simulink model "RigidJoint_Adaptive_PD"  (R2019b)
settings: Solver=VariableStepAuto  StartTime=0.0  StopTime=10  RelTol=1e-3
libraries: simulink x6
settings Model: Creator=USER  LastModifiedBy=USER

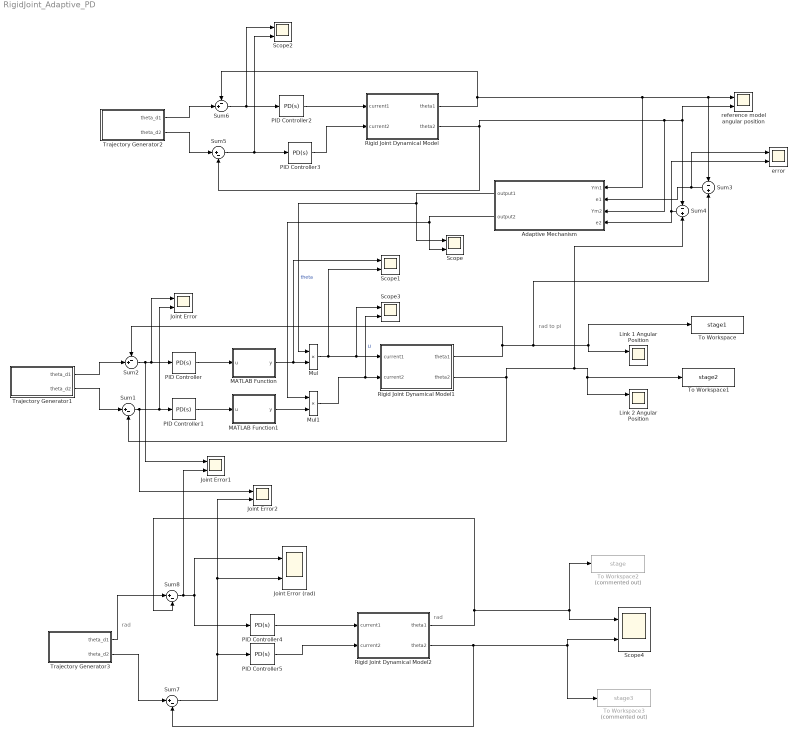
== system RigidJoint_Adaptive_PD ==
  note: rad to pi
  note: rad
  note: rad
  Adaptive Mechanism : Subsystem
  Joint Error : Scope  NumInputPorts=2
  Joint Error (rad) : Scope  NumInputPorts=2
  Joint Error1 : Scope  NumInputPorts=2
  Joint Error2 : Scope  NumInputPorts=2
  Link 1 Angular Position : Scope  NumInputPorts=2
  Link 2 Angular Position : Scope  NumInputPorts=2
  MATLAB Function : MATLAB Function  TreatAsAtomicUnit=on
  MATLAB Function1 : MATLAB Function  TreatAsAtomicUnit=on
  Mul : Product
  Mul1 : Product
  PID Controller : simulink/Continuous/PID Controller  Controller=PD  Form=Parallel  TimeDomain=Continuous-time  SampleTime=-1  IntegratorMethod=Forward Euler  FilterMethod=Forward Euler  ControllerParametersSource=internal  P=3  I=0.00248207984793386  D=0.6  UseFilter=on  N=100  TunerSelectOption=Transfer Function Based (PID Tuner App)  InitialConditionSource=internal  InitialConditionForIntegrator=0  InitialConditionForFilter=0  DifferentiatorICPrevScaledInput=0  ExternalReset=none  TrackingMode=off  Kt=1  LimitOutput=off  UpperSaturationLimit=inf  LowerSaturationLimit=-inf  LinearizeAsGain=on  AntiWindupMode=none  Kb=1  POutMin=[]  POutMax=[]  IOutMin=[]  IOutMax=[]  DOutMin=[]  DOutMax=[]  NOutMin=[]  NOutMax=[]  SumOutMin=[]  SumOutMax=[]  SaturationOutMin=[]  SaturationOutMax=[]  PParamMin=[]  PParamMax=[]  IParamMin=[]  IParamMax=[]  DParamMin=[]  DParamMax=[]  NParamMin=[]  NParamMax=[]  KbParamMin=[]  KbParamMax=[]  KtParamMin=[]  KtParamMax=[]  KbOutMin=[]  KbOutMax=[]  KtOutMin=[]  KtOutMax=[]  IntegratorOutMin=[]  IntegratorOutMax=[]  FilterOutMin=[]  FilterOutMax=[]  SumI1OutMin=[]  SumI1OutMax=[]  SumI2OutMin=[]  SumI2OutMax=[]  SumI3OutMin=[]  SumI3OutMax=[]  SumI4OutMin=[]  SumI4OutMax=[]  SumDOutMin=[]  SumDOutMax=[]  DifferentiatorOutMin=[]  DifferentiatorOutMax=[]  FilterDiffOutCoefMin=[]  FilterDiffOutCoefMax=[]  ReciprocalOutMin=[]  ReciprocalOutMax=[]  SumDenOutMin=[]  SumDenOutMax=[]  SumNumOutMin=[]  SumNumOutMax=[]  DivideOutMin=[]  DivideOutMax=[]  IntegratorContinuousStateAttributes=''  IntegratorStateMustResolveToSignalObject=off  IntegratorRTWStateStorageClass=Auto  FilterContinuousStateAttributes=''  FilterStateMustResolveToSignalObject=off  FilterRTWStateStorageClass=Auto  ParallelPVariant=InternalParameters  IdealPVariant=Disabled  IVariant=Disabled  DVariant=InternalParameters  IntegratorVariant=Disabled  SatVariant=Disabled  AWVariant=Disabled  PCopyVariant=Disabled  TRVariant=Disabled  FdbkBlocksVariant=Forward  IdealPFdbkVariant=Disabled  SatFdbkVariant=Disabled  DerivativeFilterVariant=ContFilter  NVariant=InternalParameters  NCopyVariant=Disabled  FilterICVariant=InternalICsFilter  IntegratorICVariant=Disabled  ExternalResetVariant=Disabled  TRSumVariant=Passthrough  SumFdbkVariant=Disabled  SumVariant=Sum_PD
  PID Controller1 : simulink/Continuous/PID Controller  Controller=PD  Form=Parallel  TimeDomain=Continuous-time  SampleTime=-1  IntegratorMethod=Forward Euler  FilterMethod=Forward Euler  ControllerParametersSource=internal  P=8  I=0.00248207984793386  D=0.8  UseFilter=on  N=100  TunerSelectOption=Transfer Function Based (PID Tuner App)  InitialConditionSource=internal  InitialConditionForIntegrator=0  InitialConditionForFilter=0  DifferentiatorICPrevScaledInput=0  ExternalReset=none  TrackingMode=off  Kt=1  LimitOutput=off  UpperSaturationLimit=inf  LowerSaturationLimit=-inf  LinearizeAsGain=on  AntiWindupMode=none  Kb=1  POutMin=[]  POutMax=[]  IOutMin=[]  IOutMax=[]  DOutMin=[]  DOutMax=[]  NOutMin=[]  NOutMax=[]  SumOutMin=[]  SumOutMax=[]  SaturationOutMin=[]  SaturationOutMax=[]  PParamMin=[]  PParamMax=[]  IParamMin=[]  IParamMax=[]  DParamMin=[]  DParamMax=[]  NParamMin=[]  NParamMax=[]  KbParamMin=[]  KbParamMax=[]  KtParamMin=[]  KtParamMax=[]  KbOutMin=[]  KbOutMax=[]  KtOutMin=[]  KtOutMax=[]  IntegratorOutMin=[]  IntegratorOutMax=[]  FilterOutMin=[]  FilterOutMax=[]  SumI1OutMin=[]  SumI1OutMax=[]  SumI2OutMin=[]  SumI2OutMax=[]  SumI3OutMin=[]  SumI3OutMax=[]  SumI4OutMin=[]  SumI4OutMax=[]  SumDOutMin=[]  SumDOutMax=[]  DifferentiatorOutMin=[]  DifferentiatorOutMax=[]  FilterDiffOutCoefMin=[]  FilterDiffOutCoefMax=[]  ReciprocalOutMin=[]  ReciprocalOutMax=[]  SumDenOutMin=[]  SumDenOutMax=[]  SumNumOutMin=[]  SumNumOutMax=[]  DivideOutMin=[]  DivideOutMax=[]  IntegratorContinuousStateAttributes=''  IntegratorStateMustResolveToSignalObject=off  IntegratorRTWStateStorageClass=Auto  FilterContinuousStateAttributes=''  FilterStateMustResolveToSignalObject=off  FilterRTWStateStorageClass=Auto  ParallelPVariant=InternalParameters  IdealPVariant=Disabled  IVariant=Disabled  DVariant=InternalParameters  IntegratorVariant=Disabled  SatVariant=Disabled  AWVariant=Disabled  PCopyVariant=Disabled  TRVariant=Disabled  FdbkBlocksVariant=Forward  IdealPFdbkVariant=Disabled  SatFdbkVariant=Disabled  DerivativeFilterVariant=ContFilter  NVariant=InternalParameters  NCopyVariant=Disabled  FilterICVariant=InternalICsFilter  IntegratorICVariant=Disabled  ExternalResetVariant=Disabled  TRSumVariant=Passthrough  SumFdbkVariant=Disabled  SumVariant=Sum_PD
  PID Controller2 : simulink/Continuous/PID Controller  Controller=PD  Form=Parallel  TimeDomain=Continuous-time  SampleTime=-1  IntegratorMethod=Forward Euler  FilterMethod=Forward Euler  ControllerParametersSource=internal  P=3  I=0.00248207984793386  D=0.6  UseFilter=on  N=100  TunerSelectOption=Transfer Function Based (PID Tuner App)  InitialConditionSource=internal  InitialConditionForIntegrator=0  InitialConditionForFilter=0  DifferentiatorICPrevScaledInput=0  ExternalReset=none  TrackingMode=off  Kt=1  LimitOutput=off  UpperSaturationLimit=inf  LowerSaturationLimit=-inf  LinearizeAsGain=on  AntiWindupMode=none  Kb=1  POutMin=[]  POutMax=[]  IOutMin=[]  IOutMax=[]  DOutMin=[]  DOutMax=[]  NOutMin=[]  NOutMax=[]  SumOutMin=[]  SumOutMax=[]  SaturationOutMin=[]  SaturationOutMax=[]  PParamMin=[]  PParamMax=[]  IParamMin=[]  IParamMax=[]  DParamMin=[]  DParamMax=[]  NParamMin=[]  NParamMax=[]  KbParamMin=[]  KbParamMax=[]  KtParamMin=[]  KtParamMax=[]  KbOutMin=[]  KbOutMax=[]  KtOutMin=[]  KtOutMax=[]  IntegratorOutMin=[]  IntegratorOutMax=[]  FilterOutMin=[]  FilterOutMax=[]  SumI1OutMin=[]  SumI1OutMax=[]  SumI2OutMin=[]  SumI2OutMax=[]  SumI3OutMin=[]  SumI3OutMax=[]  SumI4OutMin=[]  SumI4OutMax=[]  SumDOutMin=[]  SumDOutMax=[]  DifferentiatorOutMin=[]  DifferentiatorOutMax=[]  FilterDiffOutCoefMin=[]  FilterDiffOutCoefMax=[]  ReciprocalOutMin=[]  ReciprocalOutMax=[]  SumDenOutMin=[]  SumDenOutMax=[]  SumNumOutMin=[]  SumNumOutMax=[]  DivideOutMin=[]  DivideOutMax=[]  IntegratorContinuousStateAttributes=''  IntegratorStateMustResolveToSignalObject=off  IntegratorRTWStateStorageClass=Auto  FilterContinuousStateAttributes=''  FilterStateMustResolveToSignalObject=off  FilterRTWStateStorageClass=Auto  ParallelPVariant=InternalParameters  IdealPVariant=Disabled  IVariant=Disabled  DVariant=InternalParameters  IntegratorVariant=Disabled  SatVariant=Disabled  AWVariant=Disabled  PCopyVariant=Disabled  TRVariant=Disabled  FdbkBlocksVariant=Forward  IdealPFdbkVariant=Disabled  SatFdbkVariant=Disabled  DerivativeFilterVariant=ContFilter  NVariant=InternalParameters  NCopyVariant=Disabled  FilterICVariant=InternalICsFilter  IntegratorICVariant=Disabled  ExternalResetVariant=Disabled  TRSumVariant=Passthrough  SumFdbkVariant=Disabled  SumVariant=Sum_PD
  PID Controller3 : simulink/Continuous/PID Controller  Controller=PD  Form=Parallel  TimeDomain=Continuous-time  SampleTime=-1  IntegratorMethod=Forward Euler  FilterMethod=Forward Euler  ControllerParametersSource=internal  P=8  I=0.00248207984793386  D=0.8  UseFilter=on  N=100  TunerSelectOption=Transfer Function Based (PID Tuner App)  InitialConditionSource=internal  InitialConditionForIntegrator=0  InitialConditionForFilter=0  DifferentiatorICPrevScaledInput=0  ExternalReset=none  TrackingMode=off  Kt=1  LimitOutput=off  UpperSaturationLimit=inf  LowerSaturationLimit=-inf  LinearizeAsGain=on  AntiWindupMode=none  Kb=1  POutMin=[]  POutMax=[]  IOutMin=[]  IOutMax=[]  DOutMin=[]  DOutMax=[]  NOutMin=[]  NOutMax=[]  SumOutMin=[]  SumOutMax=[]  SaturationOutMin=[]  SaturationOutMax=[]  PParamMin=[]  PParamMax=[]  IParamMin=[]  IParamMax=[]  DParamMin=[]  DParamMax=[]  NParamMin=[]  NParamMax=[]  KbParamMin=[]  KbParamMax=[]  KtParamMin=[]  KtParamMax=[]  KbOutMin=[]  KbOutMax=[]  KtOutMin=[]  KtOutMax=[]  IntegratorOutMin=[]  IntegratorOutMax=[]  FilterOutMin=[]  FilterOutMax=[]  SumI1OutMin=[]  SumI1OutMax=[]  SumI2OutMin=[]  SumI2OutMax=[]  SumI3OutMin=[]  SumI3OutMax=[]  SumI4OutMin=[]  SumI4OutMax=[]  SumDOutMin=[]  SumDOutMax=[]  DifferentiatorOutMin=[]  DifferentiatorOutMax=[]  FilterDiffOutCoefMin=[]  FilterDiffOutCoefMax=[]  ReciprocalOutMin=[]  ReciprocalOutMax=[]  SumDenOutMin=[]  SumDenOutMax=[]  SumNumOutMin=[]  SumNumOutMax=[]  DivideOutMin=[]  DivideOutMax=[]  IntegratorContinuousStateAttributes=''  IntegratorStateMustResolveToSignalObject=off  IntegratorRTWStateStorageClass=Auto  FilterContinuousStateAttributes=''  FilterStateMustResolveToSignalObject=off  FilterRTWStateStorageClass=Auto  ParallelPVariant=InternalParameters  IdealPVariant=Disabled  IVariant=Disabled  DVariant=InternalParameters  IntegratorVariant=Disabled  SatVariant=Disabled  AWVariant=Disabled  PCopyVariant=Disabled  TRVariant=Disabled  FdbkBlocksVariant=Forward  IdealPFdbkVariant=Disabled  SatFdbkVariant=Disabled  DerivativeFilterVariant=ContFilter  NVariant=InternalParameters  NCopyVariant=Disabled  FilterICVariant=InternalICsFilter  IntegratorICVariant=Disabled  ExternalResetVariant=Disabled  TRSumVariant=Passthrough  SumFdbkVariant=Disabled  SumVariant=Sum_PD
  PID Controller4 : simulink/Continuous/PID Controller  Controller=PD  Form=Parallel  TimeDomain=Continuous-time  SampleTime=-1  IntegratorMethod=Forward Euler  FilterMethod=Forward Euler  ControllerParametersSource=internal  P=3  I=0.00248207984793386  D=0.6  UseFilter=on  N=100  TunerSelectOption=Transfer Function Based (PID Tuner App)  InitialConditionSource=internal  InitialConditionForIntegrator=0  InitialConditionForFilter=0  DifferentiatorICPrevScaledInput=0  ExternalReset=none  TrackingMode=off  Kt=1  LimitOutput=off  UpperSaturationLimit=inf  LowerSaturationLimit=-inf  LinearizeAsGain=on  AntiWindupMode=none  Kb=1  POutMin=[]  POutMax=[]  IOutMin=[]  IOutMax=[]  DOutMin=[]  DOutMax=[]  NOutMin=[]  NOutMax=[]  SumOutMin=[]  SumOutMax=[]  SaturationOutMin=[]  SaturationOutMax=[]  PParamMin=[]  PParamMax=[]  IParamMin=[]  IParamMax=[]  DParamMin=[]  DParamMax=[]  NParamMin=[]  NParamMax=[]  KbParamMin=[]  KbParamMax=[]  KtParamMin=[]  KtParamMax=[]  KbOutMin=[]  KbOutMax=[]  KtOutMin=[]  KtOutMax=[]  IntegratorOutMin=[]  IntegratorOutMax=[]  FilterOutMin=[]  FilterOutMax=[]  SumI1OutMin=[]  SumI1OutMax=[]  SumI2OutMin=[]  SumI2OutMax=[]  SumI3OutMin=[]  SumI3OutMax=[]  SumI4OutMin=[]  SumI4OutMax=[]  SumDOutMin=[]  SumDOutMax=[]  DifferentiatorOutMin=[]  DifferentiatorOutMax=[]  FilterDiffOutCoefMin=[]  FilterDiffOutCoefMax=[]  ReciprocalOutMin=[]  ReciprocalOutMax=[]  SumDenOutMin=[]  SumDenOutMax=[]  SumNumOutMin=[]  SumNumOutMax=[]  DivideOutMin=[]  DivideOutMax=[]  IntegratorContinuousStateAttributes=''  IntegratorStateMustResolveToSignalObject=off  IntegratorRTWStateStorageClass=Auto  FilterContinuousStateAttributes=''  FilterStateMustResolveToSignalObject=off  FilterRTWStateStorageClass=Auto  ParallelPVariant=InternalParameters  IdealPVariant=Disabled  IVariant=Disabled  DVariant=InternalParameters  IntegratorVariant=Disabled  SatVariant=Disabled  AWVariant=Disabled  PCopyVariant=Disabled  TRVariant=Disabled  FdbkBlocksVariant=Forward  IdealPFdbkVariant=Disabled  SatFdbkVariant=Disabled  DerivativeFilterVariant=ContFilter  NVariant=InternalParameters  NCopyVariant=Disabled  FilterICVariant=InternalICsFilter  IntegratorICVariant=Disabled  ExternalResetVariant=Disabled  TRSumVariant=Passthrough  SumFdbkVariant=Disabled  SumVariant=Sum_PD
  PID Controller5 : simulink/Continuous/PID Controller  Controller=PD  Form=Parallel  TimeDomain=Continuous-time  SampleTime=-1  IntegratorMethod=Forward Euler  FilterMethod=Forward Euler  ControllerParametersSource=internal  P=8  I=0.00248207984793386  D=0.8  UseFilter=on  N=100  TunerSelectOption=Transfer Function Based (PID Tuner App)  InitialConditionSource=internal  InitialConditionForIntegrator=0  InitialConditionForFilter=0  DifferentiatorICPrevScaledInput=0  ExternalReset=none  TrackingMode=off  Kt=1  LimitOutput=off  UpperSaturationLimit=inf  LowerSaturationLimit=-inf  LinearizeAsGain=on  AntiWindupMode=none  Kb=1  POutMin=[]  POutMax=[]  IOutMin=[]  IOutMax=[]  DOutMin=[]  DOutMax=[]  NOutMin=[]  NOutMax=[]  SumOutMin=[]  SumOutMax=[]  SaturationOutMin=[]  SaturationOutMax=[]  PParamMin=[]  PParamMax=[]  IParamMin=[]  IParamMax=[]  DParamMin=[]  DParamMax=[]  NParamMin=[]  NParamMax=[]  KbParamMin=[]  KbParamMax=[]  KtParamMin=[]  KtParamMax=[]  KbOutMin=[]  KbOutMax=[]  KtOutMin=[]  KtOutMax=[]  IntegratorOutMin=[]  IntegratorOutMax=[]  FilterOutMin=[]  FilterOutMax=[]  SumI1OutMin=[]  SumI1OutMax=[]  SumI2OutMin=[]  SumI2OutMax=[]  SumI3OutMin=[]  SumI3OutMax=[]  SumI4OutMin=[]  SumI4OutMax=[]  SumDOutMin=[]  SumDOutMax=[]  DifferentiatorOutMin=[]  DifferentiatorOutMax=[]  FilterDiffOutCoefMin=[]  FilterDiffOutCoefMax=[]  ReciprocalOutMin=[]  ReciprocalOutMax=[]  SumDenOutMin=[]  SumDenOutMax=[]  SumNumOutMin=[]  SumNumOutMax=[]  DivideOutMin=[]  DivideOutMax=[]  IntegratorContinuousStateAttributes=''  IntegratorStateMustResolveToSignalObject=off  IntegratorRTWStateStorageClass=Auto  FilterContinuousStateAttributes=''  FilterStateMustResolveToSignalObject=off  FilterRTWStateStorageClass=Auto  ParallelPVariant=InternalParameters  IdealPVariant=Disabled  IVariant=Disabled  DVariant=InternalParameters  IntegratorVariant=Disabled  SatVariant=Disabled  AWVariant=Disabled  PCopyVariant=Disabled  TRVariant=Disabled  FdbkBlocksVariant=Forward  IdealPFdbkVariant=Disabled  SatFdbkVariant=Disabled  DerivativeFilterVariant=ContFilter  NVariant=InternalParameters  NCopyVariant=Disabled  FilterICVariant=InternalICsFilter  IntegratorICVariant=Disabled  ExternalResetVariant=Disabled  TRSumVariant=Passthrough  SumFdbkVariant=Disabled  SumVariant=Sum_PD
  Rigid Joint Dynamical Model : Subsystem
  Rigid Joint Dynamical Model1 : Subsystem
  Rigid Joint Dynamical Model2 : Subsystem
  Scope{,1..4} (5 alike) : Scope  NumInputPorts=2
  Sum{1,5,7..8} (4 alike) : Sum  Inputs=|+-
  Sum2 : Sum  Inputs=-+|
  Sum3 : Sum  Inputs=-|+
  Sum4 : Sum  Inputs=-|+
  Sum6 : Sum  Inputs=-+|
  To Workspace : ToWorkspace  VariableName=stage1  SaveFormat=Timeseries  SampleTime=-1
  To Workspace1 : ToWorkspace  VariableName=stage2  SaveFormat=Timeseries  SampleTime=-1
  To Workspace2 : ToWorkspace  Commented=on  VariableName=stage  SaveFormat=Timeseries  SampleTime=-1
  To Workspace3 : ToWorkspace  Commented=on  VariableName=stage3  SaveFormat=Timeseries  SampleTime=-1
  Trajectory Generator1 : MATLAB Function  TreatAsAtomicUnit=on
  Trajectory Generator2 : MATLAB Function  TreatAsAtomicUnit=on
  Trajectory Generator3 : MATLAB Function  TreatAsAtomicUnit=on
  error : Scope  NumInputPorts=2
  reference model angular position : Scope  NumInputPorts=2
  wires:
  PID Controller3/1 -> Rigid Joint Dynamical Model/2("current2 ")
  Trajectory Generator2/2(theta_d2) -> Sum5/1
  Mul/1 -> Scope3/1, Rigid Joint Dynamical Model1/1(current1), Scope1/2
  PID Controller1/1 -> MATLAB Function1/1(u)
  Trajectory Generator2/1(theta_d1) -> Sum6/2
  Sum1/1 -> Joint Error2/1, PID Controller1/1, Joint Error/2
  Trajectory Generator1/2(theta_d2) -> Sum1/1
  PID Controller2/1 -> Rigid Joint Dynamical Model/1(current1)
  Sum6/1 -> Scope2/1, PID Controller2/1
  Adaptive Mechanism/1(output1) -> Scope/1, Mul/1  "theta"
  PID Controller/1 -> MATLAB Function/1(u)
  Rigid Joint Dynamical Model/2(theta2) -> Sum4/1, reference model angular position/2, Adaptive Mechanism/3(Ym2), Sum5/2
  Adaptive Mechanism/2(output2) -> Scope/2, Mul1/1
  Sum2/1 -> Joint Error1/1, Joint Error/1, PID Controller/1
  Rigid Joint Dynamical Model1/2(theta2) -> Sum4/2, Link 2 Angular Position/1, To Workspace1/1, Sum1/2
  Sum4/1 -> error/2, Adaptive Mechanism/4(e2)
  Sum3/1 -> Adaptive Mechanism/2(e1), error/1
  Rigid Joint Dynamical Model1/1(theta1) -> Link 1 Angular Position/1, To Workspace/1, Sum3/2, Sum2/1
  Mul1/1 -> Scope3/2, Rigid Joint Dynamical Model1/2("current2 ")  "U"
  Rigid Joint Dynamical Model/1(theta1) -> Adaptive Mechanism/1(Ym1), Sum3/1, reference model angular position/1, Sum6/1
  Trajectory Generator1/1(theta_d1) -> Sum2/2
  Sum5/1 -> Scope2/2, PID Controller3/1
  MATLAB Function/1(y) -> Scope1/1, Mul/2
  MATLAB Function1/1(y) -> Mul1/2
  Trajectory Generator3/1(theta_d1) -> Sum8/1
  Sum8/1 -> Joint Error1/2, Joint Error (rad)/1, PID Controller4/1
  Sum7/1 -> Joint Error2/2, Joint Error (rad)/2, PID Controller5/1
  Rigid Joint Dynamical Model2/1(theta1) -> Scope4/1, To Workspace2/1, Sum8/2
  Trajectory Generator3/2(theta_d2) -> Sum7/1
  PID Controller4/1 -> Rigid Joint Dynamical Model2/1(current1)
  PID Controller5/1 -> Rigid Joint Dynamical Model2/2("current2 ")
  Rigid Joint Dynamical Model2/2(theta2) -> To Workspace3/1, Scope4/2, Sum7/2

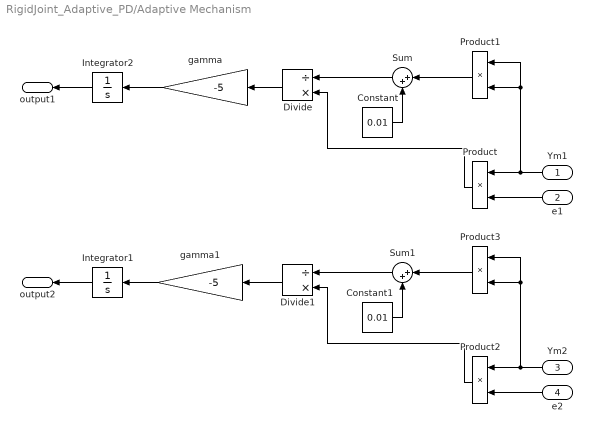
== system RigidJoint_Adaptive_PD/Adaptive Mechanism ==
  Ym1 : Inport
  e1 : Inport  Port=2
  Ym2 : Inport  Port=3
  e2 : Inport  Port=4
  Constant : Constant  Value=0.01
  Constant1 : Constant  Value=0.01
  Divide : Product  Inputs=/*
  Divide1 : Product  Inputs=/*
  Integrator1 : Integrator  InitialCondition=1
  Integrator2 : Integrator  InitialCondition=1
  Product{,1..3} (4 alike) : Product
  Sum : Sum  Inputs=|++
  Sum1 : Sum  Inputs=|++
  gamma : Gain  Gain=-5
  gamma1 : Gain  Gain=-5
  output1 : Outport  VectorParamsAs1DForOutWhenUnconnected=off
  output2 : Outport  Port=2  VectorParamsAs1DForOutWhenUnconnected=off
  wires:
  e2/1 -> Product2/2
  Ym2/1 -> Product3/1, Product3/2, Product2/1
  Product2/1 -> Divide1/2
  Constant1/1 -> Sum1/2
  Sum1/1 -> Divide1/1
  Product3/1 -> Sum1/1
  Divide1/1 -> gamma1/1
  Integrator1/1 -> output2/1
  gamma1/1 -> Integrator1/1
  Product1/1 -> Sum/1
  Integrator2/1 -> output1/1
  Divide/1 -> gamma/1
  gamma/1 -> Integrator2/1
  Constant/1 -> Sum/2
  Product/1 -> Divide/2
  Sum/1 -> Divide/1
  Ym1/1 -> Product1/1, Product1/2, Product/1
  e1/1 -> Product/2

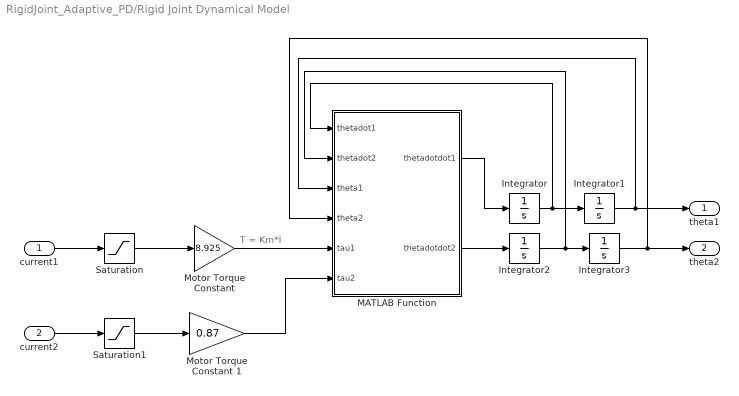
== system RigidJoint_Adaptive_PD/Rigid Joint Dynamical Model ==
  note: T = Km*I
  current1 : Inport
  "current2 " : Inport  Port=2
  Integrator{,1..3} (4 alike) : Integrator
  MATLAB Function : MATLAB Function  TreatAsAtomicUnit=on
  "Motor Torque Constant " : Gain  Gain=8.925
  Motor Torque Constant 1 : Gain  Gain=0.87
  Saturation : Saturate  UpperLimit=1  LowerLimit=-1
  Saturation1 : Saturate
  theta1 : Outport
  theta2 : Outport  Port=2
  wires:
  Integrator1/1 -> MATLAB Function/3(theta1), theta1/1
  "Motor Torque Constant "/1 -> MATLAB Function/5(tau1)
  Integrator/1 -> MATLAB Function/1(thetadot1), Integrator1/1
  MATLAB Function/1(thetadotdot1) -> Integrator/1
  Saturation/1 -> "Motor Torque Constant "/1
  current1/1 -> Saturation/1
  MATLAB Function/2(thetadotdot2) -> Integrator2/1
  Integrator2/1 -> MATLAB Function/2(thetadot2), Integrator3/1
  Integrator3/1 -> MATLAB Function/4(theta2), theta2/1
  Motor Torque Constant 1/1 -> MATLAB Function/6(tau2)
  "current2 "/1 -> Saturation1/1
  Saturation1/1 -> Motor Torque Constant 1/1

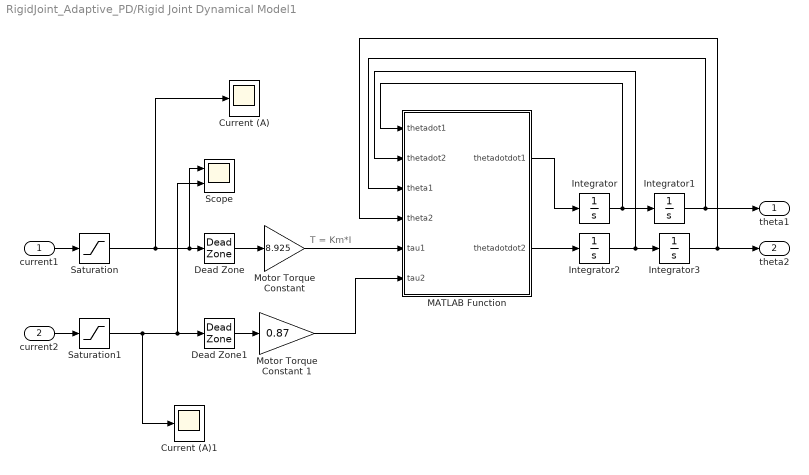
== system RigidJoint_Adaptive_PD/Rigid Joint Dynamical Model1 ==
  note: T = Km*I
  current1 : Inport
  "current2 " : Inport  Port=2
  Current (A) : Scope
  Current (A)1 : Scope
  Dead Zone : DeadZone  LowerValue=-0.15  UpperValue=0.15  SaturateOnIntegerOverflow=on
  Dead Zone1 : DeadZone  LowerValue=-0.15  UpperValue=0.15  SaturateOnIntegerOverflow=on
  Integrator{,1..3} (4 alike) : Integrator
  MATLAB Function : MATLAB Function  TreatAsAtomicUnit=on
  "Motor Torque Constant " : Gain  Gain=8.925
  Motor Torque Constant 1 : Gain  Gain=0.87
  Saturation : Saturate  UpperLimit=1  LowerLimit=-1
  Saturation1 : Saturate
  Scope : Scope  NumInputPorts=2
  theta1 : Outport
  theta2 : Outport  Port=2
  wires:
  Integrator1/1 -> MATLAB Function/3(theta1), theta1/1
  "Motor Torque Constant "/1 -> MATLAB Function/5(tau1)
  Integrator/1 -> MATLAB Function/1(thetadot1), Integrator1/1
  MATLAB Function/1(thetadotdot1) -> Integrator/1
  Saturation/1 -> Current (A)/1, Scope/1, Dead Zone/1
  current1/1 -> Saturation/1
  MATLAB Function/2(thetadotdot2) -> Integrator2/1
  Integrator2/1 -> MATLAB Function/2(thetadot2), Integrator3/1
  Integrator3/1 -> MATLAB Function/4(theta2), theta2/1
  Motor Torque Constant 1/1 -> MATLAB Function/6(tau2)
  "current2 "/1 -> Saturation1/1
  Saturation1/1 -> Current (A)1/1, Dead Zone1/1, Scope/2
  Dead Zone/1 -> "Motor Torque Constant "/1
  Dead Zone1/1 -> Motor Torque Constant 1/1

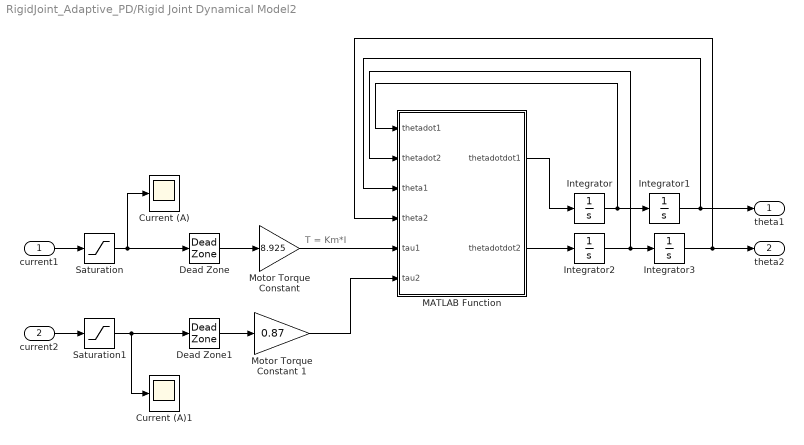
== system RigidJoint_Adaptive_PD/Rigid Joint Dynamical Model2 ==
  note: T = Km*I
  current1 : Inport
  "current2 " : Inport  Port=2
  Current (A) : Scope
  Current (A)1 : Scope
  Dead Zone : DeadZone  LowerValue=-0.2  UpperValue=0.2  SaturateOnIntegerOverflow=on
  Dead Zone1 : DeadZone  LowerValue=-0.15  UpperValue=0.15  SaturateOnIntegerOverflow=on
  Integrator{,1..3} (4 alike) : Integrator
  MATLAB Function : MATLAB Function  TreatAsAtomicUnit=on
  "Motor Torque Constant " : Gain  Gain=8.925
  Motor Torque Constant 1 : Gain  Gain=0.87
  Saturation : Saturate  UpperLimit=1  LowerLimit=-1
  Saturation1 : Saturate
  theta1 : Outport
  theta2 : Outport  Port=2
  wires:
  Integrator1/1 -> MATLAB Function/3(theta1), theta1/1
  "Motor Torque Constant "/1 -> MATLAB Function/5(tau1)
  Integrator/1 -> MATLAB Function/1(thetadot1), Integrator1/1
  MATLAB Function/1(thetadotdot1) -> Integrator/1
  current1/1 -> Saturation/1
  MATLAB Function/2(thetadotdot2) -> Integrator2/1
  Integrator2/1 -> MATLAB Function/2(thetadot2), Integrator3/1
  Integrator3/1 -> MATLAB Function/4(theta2), theta2/1
  Motor Torque Constant 1/1 -> MATLAB Function/6(tau2)
  "current2 "/1 -> Saturation1/1
  Saturation1/1 -> Dead Zone1/1, Current (A)1/1
  Saturation/1 -> Dead Zone/1, Current (A)/1
  Dead Zone/1 -> "Motor Torque Constant "/1
  Dead Zone1/1 -> Motor Torque Constant 1/1

== matlab function RigidJoint_Adaptive_PD/Trajectory Generator1 ==
  data: theta_d1 output; theta_d2 output
function [theta_d1,theta_d2]  = fcn
theta_start1 = 0;
theta_start2 = 0;
theta_end1 = pi/4;
theta_end2 = pi/4;
theta_d1 = theta_start1 + (theta_end1-theta_start1);
theta_d2 = theta_start2 + (theta_end2-theta_start2);

== matlab function RigidJoint_Adaptive_PD/Rigid Joint Dynamical Model1/MATLAB Function ==
  data: thetadot1 input; thetadotdot1 output; thetadot2 input; theta1 input; theta2 input; tau1 input; thetadotdot2 output; tau2 input
function [thetadotdot1,thetadotdot2] = fcn(thetadot1,thetadot2,theta1,theta2,tau1,tau2)
%y is thetadotdot
tau = [tau1;tau2];
%Veltman Thesis Values
% m1 = 0.5; 
% m2 = 1;
% L1 = 0.343;
% L2 = 0.267;
% Lc1 = 0.2;
% Lc2 = 0.25;
% I1 = 0.01;
% I2 = 0.01;
% B1 = 0.070364;
% B2 = 0.028211;

%Electrical School values
m1 =  1.51 ; 
m2 = 0.87326;
L1 = 0.343;
L2 = 0.267;
Lc1 = 0.1590;
Lc2 = 0.0550;
I1 = 0.0392;
I2 = 0.0081;
B1 = 0.070364;
B2 = 0.028211;


M11 = I2+I1+m2*((L1^2)+(Lc2^2)+2*L1*Lc2*cos(theta2))+m1*(Lc1^2);
M12 = I2+m2*(Lc2^2)+L1*Lc2*m2*cos(theta2);
M21 = M12;
M22 = I2+m2*(Lc2^2);

M = [M11 M12;
     M21 M22];
 
C11 = -m2*L1*Lc2*sin(theta2)*thetadot2;
C12 = -m2*L1*Lc2*sin(theta2)*thetadot2-m2*L1*Lc2*sin(theta2)*thetadot1;
C21 = m2*L1*Lc2*sin(theta2)*thetadot1;
C22 = 0;

C = [C11 C12;
     C21 C22];

C1 = C*[thetadot1;thetadot2];
 
fv = [B1;B2];

thetadotdot = inv(M)*(tau-C1-fv);
thetadotdot1 = thetadotdot(1);
thetadotdot2 = thetadotdot(2);

== matlab function RigidJoint_Adaptive_PD/Rigid Joint Dynamical Model/MATLAB Function ==
  data: thetadot1 input; thetadotdot1 output; thetadot2 input; theta1 input; theta2 input; tau1 input; thetadotdot2 output; tau2 input
function [thetadotdot1,thetadotdot2] = fcn(thetadot1,thetadot2,theta1,theta2,tau1,tau2)
%y is thetadotdot
tau = [tau1;tau2];
%Veltman Thesis Values
% m1 = 0.5; 
% m2 = 1;
% L1 = 0.343;
% L2 = 0.267;
% Lc1 = 0.2;
% Lc2 = 0.25;
% I1 = 0.01;
% I2 = 0.01;
% B1 = 0.070364;
% B2 = 0.028211;

%Electrical School values
m1 =  1.51 ; 
m2 = 0.87326;
L1 = 0.343;
L2 = 0.267;
Lc1 = 0.1590;
Lc2 = 0.0550;
I1 = 0.0392;
I2 = 0.0081;
B1 = 0.070364;
B2 = 0.028211;


M11 = I2+I1+m2*((L1^2)+(Lc2^2)+2*L1*Lc2*cos(theta2))+m1*(Lc1^2);
M12 = I2+m2*(Lc2^2)+L1*Lc2*m2*cos(theta2);
M21 = M12;
M22 = I2+m2*(Lc2^2);

M = [M11 M12;
     M21 M22];
 
C11 = -m2*L1*Lc2*sin(theta2)*thetadot2;
C12 = -m2*L1*Lc2*sin(theta2)*thetadot2-m2*L1*Lc2*sin(theta2)*thetadot1;
C21 = m2*L1*Lc2*sin(theta2)*thetadot1;
C22 = 0;

C = [C11 C12;
     C21 C22];

C1 = C*[thetadot1;thetadot2];
 
fv = [B1;B2];

thetadotdot = inv(M)*(tau-C1-fv);
thetadotdot1 = thetadotdot(1);
thetadotdot2 = thetadotdot(2);

== matlab function RigidJoint_Adaptive_PD/Trajectory Generator2 ==
  data: theta_d1 output; theta_d2 output
function [theta_d1,theta_d2]  = fcn
theta_start1 = 0;
theta_start2 = 0;
theta_end1 = pi/4;
theta_end2 = pi/4;
theta_d1 = theta_start1 + (theta_end1-theta_start1);
theta_d2 = theta_start2 + (theta_end2-theta_start2);

== matlab function RigidJoint_Adaptive_PD/MATLAB Function ==
  data: u input; y output
function y = fcn(u)

    if (u>0) 
        y = u + 0.1; %compensate deadzone values
    elseif (u<0)
        y = u - 0.1;
    else
        y=u;
    end

== matlab function RigidJoint_Adaptive_PD/MATLAB Function1 ==
  data: u input; y output
function y = fcn(u)

    if (u>0) 
        y = u + 0.1; %compensate deadzone values
    elseif (u<0)
        y = u - 0.1;
    else
        y=u;
    end

== matlab function RigidJoint_Adaptive_PD/Rigid Joint Dynamical Model2/MATLAB Function ==
  data: thetadot1 input; thetadotdot1 output; thetadot2 input; theta1 input; theta2 input; tau1 input; thetadotdot2 output; tau2 input
function [thetadotdot1,thetadotdot2] = fcn(thetadot1,thetadot2,theta1,theta2,tau1,tau2)
%y is thetadotdot
tau = [tau1;tau2];
%Veltman Thesis Values
% m1 = 0.5; 
% m2 = 1;
% L1 = 0.343;
% L2 = 0.267;
% Lc1 = 0.2;
% Lc2 = 0.25;
% I1 = 0.01;
% I2 = 0.01;
% B1 = 0.070364;
% B2 = 0.028211;

%Electrical School values
m1 =  1.51 ; 
m2 = 0.87326;
L1 = 0.343;
L2 = 0.267;
Lc1 = 0.1590;
Lc2 = 0.0550;
I1 = 0.0392;
I2 = 0.0081;
B1 = 0.070364;
B2 = 0.028211;


M11 = I2+I1+m2*((L1^2)+(Lc2^2)+2*L1*Lc2*cos(theta2))+m1*(Lc1^2);
M12 = I2+m2*(Lc2^2)+L1*Lc2*m2*cos(theta2);
M21 = M12;
M22 = I2+m2*(Lc2^2);

M = [M11 M12;
     M21 M22];
 
C11 = -m2*L1*Lc2*sin(theta2)*thetadot2;
C12 = -m2*L1*Lc2*sin(theta2)*thetadot2-m2*L1*Lc2*sin(theta2)*thetadot1;
C21 = m2*L1*Lc2*sin(theta2)*thetadot1;
C22 = 0;

C = [C11 C12;
     C21 C22];

C1 = C*[thetadot1;thetadot2];
 
fv = [B1;B2];

thetadotdot = inv(M)*(tau-C1-fv);
thetadotdot1 = thetadotdot(1);
thetadotdot2 = thetadotdot(2);

== matlab function RigidJoint_Adaptive_PD/Trajectory Generator3 ==
  data: theta_d1 output; theta_d2 output
function [theta_d1,theta_d2]  = fcn
theta_start1 = 0;
theta_start2 = 0;
theta_end1 = pi/4;
theta_end2 = pi/4;
theta_d1 = theta_start1 + (theta_end1-theta_start1);
theta_d2 = theta_start2 + (theta_end2-theta_start2);
